simulink model "CentraInver"  (R2024b)
settings: Solver=VariableStepAuto  StartTime=0.0  StopTime=20  RelTol=1e-3
libraries: Mako_Dynamics x2
settings Model: Creator=pinto  LastModifiedBy=pinto

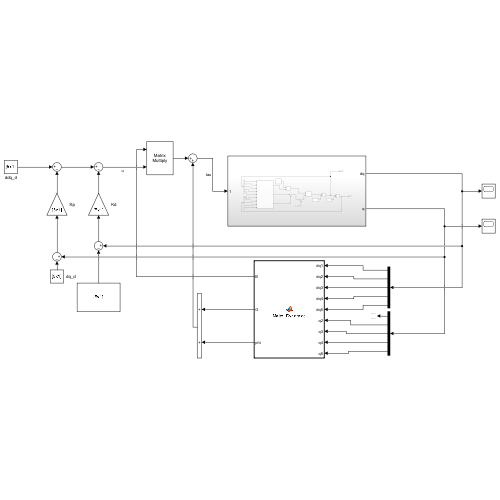
[thumbnail: Simulink's stored preview of the top-level diagram]
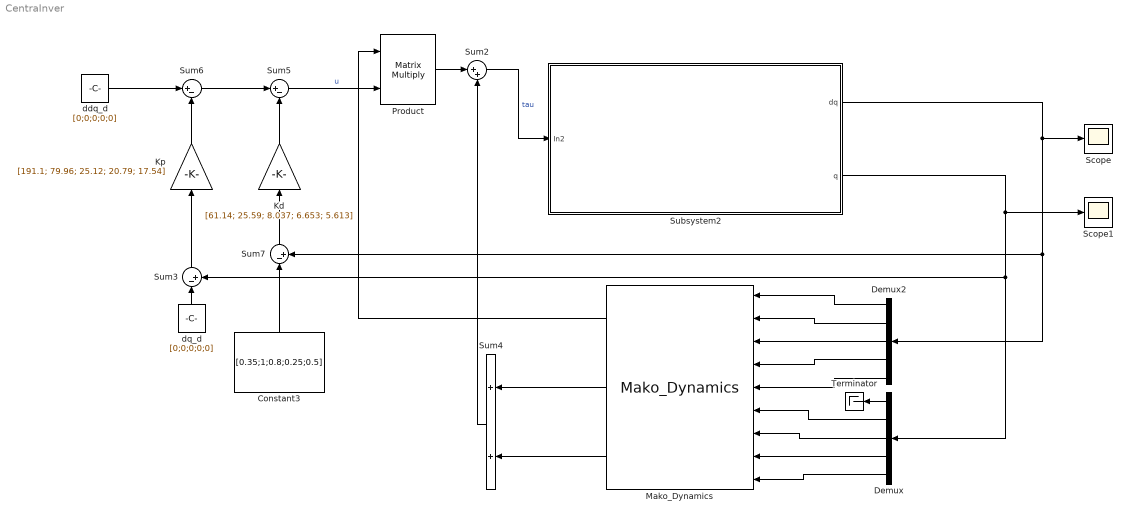
== system CentraInver ==
  Constant3 : Constant  Value=[0.35;1;0.8;0.25;0.5]
  Demux : Demux  Outputs=5
  Demux2 : Demux  Outputs=5
  Kd : Gain  Gain=[61.14; 25.59; 8.037; 6.653; 5.613]
  Kp : Gain  Gain=[191.1; 79.96; 25.12; 20.79; 17.54]
  Mako_Dynamics : Mako_Dynamics/Mako_Dynamics  SystemSampleTime=-1  VariantActivationTime=update diagram  AllowFlexibleInterface=on  Latency=0  AutoFrameSizeCalculation=off
  Product : Product  Multiplication=Matrix(*)
  Scope : Scope
  Scope1 : Scope
  Subsystem2 : Subsystem
  Sum2 : Sum  Inputs=|++
  Sum3 : Sum  Inputs=|-+
  Sum4 : Sum
  Sum5 : Sum  Inputs=|+-
  Sum6 : Sum  Inputs=|+-
  Sum7 : Sum  Inputs=|-+
  Terminator : Terminator
  ddq_d : Constant  Value=[0;0;0;0;0]
  dq_d : Constant  Value=[0;0;0;0;0]
  wires:
  Sum5/1 -> Product/2  "u"
  ddq_d/1 -> Sum6/1
  Kd/1 -> Sum5/2
  Subsystem2/2(q) -> Scope1/1, Demux/1, Sum3/2
  Sum6/1 -> Sum5/1
  Product/1 -> Sum2/1
  Kp/1 -> Sum6/2
  Sum3/1 -> Kp/1
  Constant3/1 -> Sum7/1
  Sum4/1 -> Sum2/2
  dq_d/1 -> Sum3/1
  Subsystem2/1(dq) -> Demux2/1, Sum7/2, Scope/1
  Sum7/1 -> Kd/1
  Sum2/1 -> Subsystem2/1(In2)  "tau"
  Demux2/4 -> Mako_Dynamics/4
  Demux2/1 -> Mako_Dynamics/1
  Demux2/3 -> Mako_Dynamics/3
  Demux2/2 -> Mako_Dynamics/2
  Mako_Dynamics/1 -> Product/1
  Demux2/5 -> Mako_Dynamics/5
  Mako_Dynamics/2 -> Sum4/1
  Mako_Dynamics/3 -> Sum4/2
  Demux/2 -> Mako_Dynamics/6
  Demux/3 -> Mako_Dynamics/7
  Demux/4 -> Mako_Dynamics/8
  Demux/5 -> Mako_Dynamics/9
  Demux/1 -> Terminator/1

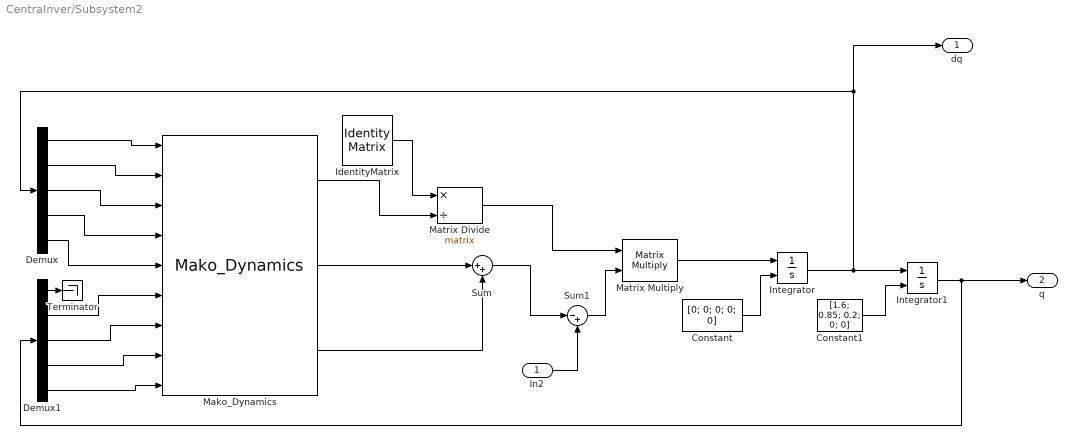
== system CentraInver/Subsystem2 ==
  In2 : Inport
  Constant : Constant  Value=[0; 0; 0; 0; 0]
  Constant1 : Constant  Value=[1.6; 0.85; 0.2; 0; 0]
  Demux : Demux  Outputs=5
  Demux1 : Demux  Outputs=5
  IdentityMatrix : IdentityMatrix
  Integrator : Integrator  InitialConditionSource=external  InitialCondition=[0.01, 0.01, 0.01]
  Integrator1 : Integrator  InitialConditionSource=external  InitialCondition=[0.01, 0.01, 0.01]
  Mako_Dynamics : Mako_Dynamics/Mako_Dynamics  SystemSampleTime=-1  VariantActivationTime=update diagram  AllowFlexibleInterface=on  Latency=0  AutoFrameSizeCalculation=off
  Matrix Divide : Product  Inputs=*/  Multiplication=Matrix(*)
  Matrix Multiply : Product  Multiplication=Matrix(*)
  Sum : Sum  Inputs=|++
  Sum1 : Sum  Inputs=|-+
  Terminator : Terminator
  dq : Outport
  q : Outport  Port=2
  wires:
  Sum/1 -> Sum1/1
  Demux/3 -> Mako_Dynamics/3
  IdentityMatrix/1 -> Matrix Divide/1
  Integrator/1 -> Integrator1/1, Demux/1, dq/1
  Matrix Multiply/1 -> Integrator/1
  Demux/4 -> Mako_Dynamics/4
  Demux/2 -> Mako_Dynamics/2
  Constant1/1 -> Integrator1/2
  Integrator1/1 -> q/1, Demux1/1
  Mako_Dynamics/1 -> Matrix Divide/2
  Matrix Divide/1 -> Matrix Multiply/1
  Constant/1 -> Integrator/2
  Sum1/1 -> Matrix Multiply/2
  Demux/1 -> Mako_Dynamics/1
  In2/1 -> Sum1/2
  Demux/5 -> Mako_Dynamics/5
  Mako_Dynamics/2 -> Sum/1
  Mako_Dynamics/3 -> Sum/2
  Demux1/2 -> Mako_Dynamics/6
  Demux1/3 -> Mako_Dynamics/7
  Demux1/4 -> Mako_Dynamics/8
  Demux1/5 -> Mako_Dynamics/9
  Demux1/1 -> Terminator/1
